simulink subsystem "Electromechanical_SubSystem"  (R2020b)
settings: Solver=VariableStepAuto  StartTime=0.0  StopTime=10.0  RelTol=1e-3
undefined symbols (not defined in the file): Fv1, Ts, ua2tau1, x0
settings Model: Creator=umberto  LastModifiedBy=Musta

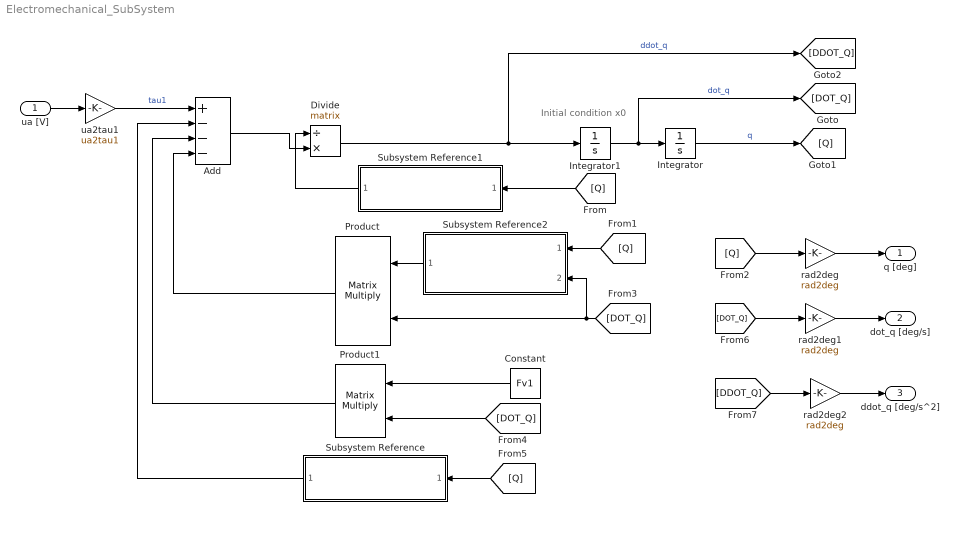
== system Electromechanical_SubSystem ==
  note: Initial condition x0
  ua [V] : Inport
  Add : Sum  Inputs=+---
  Constant : Constant  Value=Fv1  SampleTime=Ts
  Divide : Product  Inputs=/*  Multiplication=Matrix(*)
  Integrator : Integrator  InitialCondition=x0(1:2)
  Integrator1 : Integrator  InitialCondition=x0(3:end)
  Product : Product  Multiplication=Matrix(*)
  Product1 : Product  Multiplication=Matrix(*)
  Subsystem Reference : Subsystem  ReferencedSubsystem=gq_SubSystem
  Subsystem Reference1 : Subsystem  ReferencedSubsystem=Mq_SubSystem
  Subsystem Reference2 : Subsystem  ReferencedSubsystem=Cqdot_q_SubSystem
  rad2deg : Gain  Gain=rad2deg
  rad2deg1 : Gain  Gain=rad2deg
  rad2deg2 : Gain  Gain=rad2deg
  ua2tau1 : Gain  Gain=ua2tau1
  q [deg] : Outport
  dot_q [deg/s] : Outport  Port=2
  ddot_q [deg/s^2] : Outport  Port=3
  wires:
  [DOT_Q] -> rad2deg1/1
  [DDOT_Q] -> rad2deg2/1
  Integrator1/1 -> Integrator/1, [DOT_Q]  "dot_q"
  Integrator/1 -> [Q]  "q"
  Divide/1 -> Integrator1/1, [DDOT_Q]  "ddot_q"
  Subsystem Reference1/1 -> Divide/1
  Add/1 -> Divide/2
  Product1/1 -> Add/3
  [Q] -> Subsystem Reference/1
  [DOT_Q] -> Product1/2
  Constant/1 -> Product1/1
  Product/1 -> Add/4
  [DOT_Q] -> Product/2, Subsystem Reference2/2
  [Q] -> rad2deg/1
  [Q] -> Subsystem Reference2/1
  [Q] -> Subsystem Reference1/1
  Subsystem Reference2/1 -> Product/1
  Subsystem Reference/1 -> Add/2
  rad2deg2/1 -> ddot_q [deg/s^2]/1
  rad2deg1/1 -> dot_q [deg/s]/1
  rad2deg/1 -> q [deg]/1
  ua2tau1/1 -> Add/1  "tau1"
  ua [V]/1 -> ua2tau1/1
